simulink model "c00016M_harness"  (R2018a)
settings: Solver=FixedStepAuto  StartTime=0.0  StopTime=300  FixedStep=0.1  RelTol=1e-3
undefined symbols (not defined in the file): A1, hmax, PriorityTank, R1, R2, sigbuilder_block
(part 1 of 24)
settings Model: Creator=aarrieta  LastModifiedBy=umarkiegi

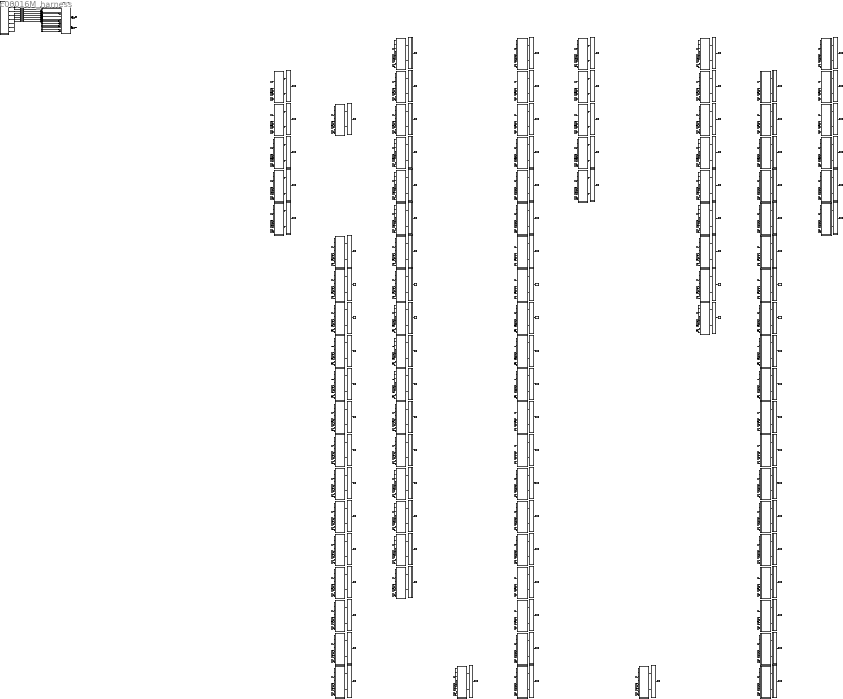
== system c00016M_harness ==
  CPSUT : Subsystem
  Eval100 : Subsystem
  Eval101 : Subsystem
  Eval102 : Subsystem
  Eval103 : Subsystem
  Eval104 : Subsystem
  Eval105 : Subsystem
  Eval106 : Subsystem
  Eval107 : Subsystem
  Eval108 : Subsystem
  Eval109 : Subsystem
  Eval110 : Subsystem
  Eval111 : Subsystem
  Eval112 : Subsystem
  Eval113 : Subsystem
  Eval114 : Subsystem
  Eval115 : Subsystem
  Eval116 : Subsystem
  Eval139 : Subsystem
  Eval140 : Subsystem
  Eval141 : Subsystem
  Eval142 : Subsystem
  Eval143 : Subsystem
  Eval144 : Subsystem
  Eval145 : Subsystem
  Eval146 : Subsystem
  Eval147 : Subsystem
  Eval148 : Subsystem
  Eval149 : Subsystem
  Eval150 : Subsystem
  Eval151 : Subsystem
  Eval152 : Subsystem
  Eval153 : Subsystem
  Eval154 : Subsystem
  Eval155 : Subsystem
  Eval156 : Subsystem
  Eval157 : Subsystem
  Eval158 : Subsystem
  Eval159 : Subsystem
  Eval160 : Subsystem
  Eval161 : Subsystem
  Eval162 : Subsystem
  Eval163 : Subsystem
  Eval164 : Subsystem
  Eval199 : Subsystem
  Eval200 : Subsystem
  Eval201 : Subsystem
  Eval202 : Subsystem
  Eval203 : Subsystem
  Eval204 : Subsystem
  Eval205 : Subsystem
  Eval206 : Subsystem
  Eval207 : Subsystem
  Eval208 : Subsystem
  Eval221 : Subsystem
  Eval222 : Subsystem
  Eval223 : Subsystem
  Eval224 : Subsystem
  Eval225 : Subsystem
  Eval226 : Subsystem
  Eval227 : Subsystem
  Eval228 : Subsystem
  Eval229 : Subsystem
  Eval230 : Subsystem
  Eval231 : Subsystem
  Eval232 : Subsystem
  Eval233 : Subsystem
  Eval234 : Subsystem
  Eval235 : Subsystem
  Eval236 : Subsystem
  Eval237 : Subsystem
  Eval238 : Subsystem
  Eval239 : Subsystem
  Eval240 : Subsystem
  Eval241 : Subsystem
  Eval242 : Subsystem
  Eval243 : Subsystem
  Eval244 : Subsystem
  Eval245 : Subsystem
  Eval61 : Subsystem
  Eval62 : Subsystem
  Eval63 : Subsystem
  Eval64 : Subsystem
  Eval65 : Subsystem
  Eval82 : Subsystem
  Eval86 : Subsystem
  Eval87 : Subsystem
  Eval88 : Subsystem
  Eval89 : Subsystem
  Eval90 : Subsystem
  Eval91 : Subsystem
  Eval92 : Subsystem
  Eval93 : Subsystem
  Eval94 : Subsystem
  Eval95 : Subsystem
  Eval96 : Subsystem
  Eval97 : Subsystem
  Eval98 : Subsystem
  Eval99 : Subsystem
  Inputs : Subsystem  Tag=STV Subsys  LoadFcn=sigbuilder_block('load');  StartFcn=sigbuilder_block('start');  StopFcn=sigbuilder_block('stop');  ClipboardFcn=sigbuilder_block('clipboard');  mask(Sigbuilder block){tuvar=[0:10]}
      mask init:
      | if ~strcmp(get_param(bdroot(gcb),'SimulationStatus'),'stopped'),tuvar = sigbuilder_block('maskInit'); end
      settings: CopyFcn=sigbuilder_block('copy');  DeleteFcn=sigbuilder_block('delete');  ModelCloseFcn=sigbuilder_block('modelClose');  PreSaveFcn=sigbuilder_block('preSave');  PauseFcn=sigbuilder_block('pause');  ContinueFcn=sigbuilder_block('continue');  NameChangeFcn=sigbuilder_block('namechange');  OpenFcn=sigbuilder_block('open',[276.75 163.5 675.75 486.75 ]);  CloseFcn=sigbuilder_block('close');
      mask Display: plot(0, 0, 100, 100,[2, 2, 32, 32, 2], [68, 8, 8, 68, 68],[32, 2], [38, 38], [32, 19, 2],[53, 60, 44], [32, 17, 17, 2],[16, 16, 31, 31]);txt = getActiveGroup(gcbh);text(2, 100, txt,'verticalAlignment', 'top');
  M062 : Subsystem
  M063 : Subsystem
  M064 : Subsystem
  M065 : Subsystem
  M066 : Subsystem
  M083 : Subsystem
  M087 : Subsystem
  M088 : Subsystem
  M089 : Subsystem
  M090 : Subsystem
  M091 : Subsystem
  M092 : Subsystem
  M093 : Subsystem
  M094 : Subsystem
  M095 : Subsystem
  M096 : Subsystem
  M097 : Subsystem
  M098 : Subsystem
  M099 : Subsystem
  M100 : Subsystem
  M101 : Subsystem
  M102 : Subsystem
  M103 : Subsystem
  M104 : Subsystem
  M105 : Subsystem
  M106 : Subsystem
  M107 : Subsystem
  M108 : Subsystem
  M109 : Subsystem
  M110 : Subsystem
  M111 : Subsystem
  M112 : Subsystem
  M113 : Subsystem
  M114 : Subsystem
  M115 : Subsystem
  M116 : Subsystem
  M117 : Subsystem
  M140 : Subsystem
  M141 : Subsystem
  M142 : Subsystem
  M143 : Subsystem
  M144 : Subsystem
  M145 : Subsystem
  M146 : Subsystem
  M147 : Subsystem
  M148 : Subsystem
  M149 : Subsystem
  M150 : Subsystem
  M151 : Subsystem
  M152 : Subsystem
  M153 : Subsystem
  M154 : Subsystem
  M155 : Subsystem
  M156 : Subsystem
  M157 : Subsystem
  M158 : Subsystem
  M159 : Subsystem
  M160 : Subsystem
  M161 : Subsystem
  M162 : Subsystem
  M163 : Subsystem
  M164 : Subsystem
  M165 : Subsystem
  M200 : Subsystem
  M201 : Subsystem
  M202 : Subsystem
  M203 : Subsystem
  M204 : Subsystem
  M205 : Subsystem
  M206 : Subsystem
  M207 : Subsystem
  M208 : Subsystem
  M209 : Subsystem
  M222 : Subsystem
  M223 : Subsystem
  M224 : Subsystem
  M225 : Subsystem
  M226 : Subsystem
  M227 : Subsystem
  M228 : Subsystem
  M229 : Subsystem
  M230 : Subsystem
  M231 : Subsystem
  M232 : Subsystem
  M233 : Subsystem
  M234 : Subsystem
  M235 : Subsystem
  M236 : Subsystem
  M237 : Subsystem
  M238 : Subsystem
  M239 : Subsystem
  M240 : Subsystem
  M241 : Subsystem
  M242 : Subsystem
  M243 : Subsystem
  M244 : Subsystem
  M245 : Subsystem
  M246 : Subsystem
  To Workspace100 : ToWorkspace  VariableName=mutant101  SampleTime=-1
  To Workspace101 : ToWorkspace  VariableName=mutant102  SampleTime=-1
  To Workspace102 : ToWorkspace  VariableName=mutant103  SampleTime=-1
  To Workspace103 : ToWorkspace  VariableName=mutant104  SampleTime=-1
  To Workspace104 : ToWorkspace  VariableName=mutant105  SampleTime=-1
  To Workspace105 : ToWorkspace  VariableName=mutant106  SampleTime=-1
  To Workspace106 : ToWorkspace  VariableName=mutant107  SampleTime=-1
  To Workspace107 : ToWorkspace  VariableName=mutant108  SampleTime=-1
  To Workspace108 : ToWorkspace  VariableName=mutant109  SampleTime=-1
  To Workspace109 : ToWorkspace  VariableName=mutant110  SampleTime=-1
  To Workspace110 : ToWorkspace  VariableName=mutant111  SampleTime=-1
  To Workspace111 : ToWorkspace  VariableName=mutant112  SampleTime=-1
  To Workspace112 : ToWorkspace  VariableName=mutant113  SampleTime=-1
  To Workspace113 : ToWorkspace  VariableName=mutant114  SampleTime=-1
  To Workspace114 : ToWorkspace  VariableName=mutant115  SampleTime=-1
  To Workspace115 : ToWorkspace  VariableName=mutant116  SampleTime=-1
  To Workspace116 : ToWorkspace  VariableName=mutant117  SampleTime=-1
  To Workspace139 : ToWorkspace  VariableName=mutant140  SampleTime=-1
  To Workspace140 : ToWorkspace  VariableName=mutant141  SampleTime=-1
  To Workspace141 : ToWorkspace  VariableName=mutant142  SampleTime=-1
  To Workspace142 : ToWorkspace  VariableName=mutant143  SampleTime=-1
  To Workspace143 : ToWorkspace  VariableName=mutant144  SampleTime=-1
  To Workspace144 : ToWorkspace  VariableName=mutant145  SampleTime=-1
  To Workspace145 : ToWorkspace  VariableName=mutant146  SampleTime=-1
  To Workspace146 : ToWorkspace  VariableName=mutant147  SampleTime=-1
  To Workspace147 : ToWorkspace  VariableName=mutant148  SampleTime=-1
  To Workspace148 : ToWorkspace  VariableName=mutant149  SampleTime=-1
  To Workspace149 : ToWorkspace  VariableName=mutant150  SampleTime=-1
  To Workspace150 : ToWorkspace  VariableName=mutant151  SampleTime=-1
  To Workspace151 : ToWorkspace  VariableName=mutant152  SampleTime=-1
  To Workspace152 : ToWorkspace  VariableName=mutant153  SampleTime=-1
  To Workspace153 : ToWorkspace  VariableName=mutant154  SampleTime=-1
  To Workspace154 : ToWorkspace  VariableName=mutant155  SampleTime=-1
  To Workspace155 : ToWorkspace  VariableName=mutant156  SampleTime=-1
  To Workspace156 : ToWorkspace  VariableName=mutant157  SampleTime=-1
  To Workspace157 : ToWorkspace  VariableName=mutant158  SampleTime=-1
  To Workspace158 : ToWorkspace  VariableName=mutant159  SampleTime=-1
  To Workspace159 : ToWorkspace  VariableName=mutant160  SampleTime=-1
  To Workspace160 : ToWorkspace  VariableName=mutant161  SampleTime=-1
  To Workspace161 : ToWorkspace  VariableName=mutant162  SampleTime=-1
  To Workspace162 : ToWorkspace  VariableName=mutant163  SampleTime=-1
  To Workspace163 : ToWorkspace  VariableName=mutant164  SampleTime=-1
  To Workspace164 : ToWorkspace  VariableName=mutant165  SampleTime=-1
  To Workspace199 : ToWorkspace  VariableName=mutant200  SampleTime=-1
  To Workspace200 : ToWorkspace  VariableName=mutant201  SampleTime=-1
  To Workspace201 : ToWorkspace  VariableName=mutant202  SampleTime=-1
  To Workspace202 : ToWorkspace  VariableName=mutant203  SampleTime=-1
  To Workspace203 : ToWorkspace  VariableName=mutant204  SampleTime=-1
  To Workspace204 : ToWorkspace  VariableName=mutant205  SampleTime=-1
  To Workspace205 : ToWorkspace  VariableName=mutant206  SampleTime=-1
  To Workspace206 : ToWorkspace  VariableName=mutant207  SampleTime=-1
  To Workspace207 : ToWorkspace  VariableName=mutant208  SampleTime=-1
  To Workspace208 : ToWorkspace  VariableName=mutant209  SampleTime=-1
  To Workspace221 : ToWorkspace  VariableName=mutant222  SampleTime=-1
  To Workspace222 : ToWorkspace  VariableName=mutant223  SampleTime=-1
  To Workspace223 : ToWorkspace  VariableName=mutant224  SampleTime=-1
  To Workspace224 : ToWorkspace  VariableName=mutant225  SampleTime=-1
  To Workspace225 : ToWorkspace  VariableName=mutant226  SampleTime=-1
  To Workspace226 : ToWorkspace  VariableName=mutant227  SampleTime=-1
  To Workspace227 : ToWorkspace  VariableName=mutant228  SampleTime=-1
  To Workspace228 : ToWorkspace  VariableName=mutant229  SampleTime=-1
  To Workspace229 : ToWorkspace  VariableName=mutant230  SampleTime=-1
  To Workspace230 : ToWorkspace  VariableName=mutant231  SampleTime=-1
  To Workspace231 : ToWorkspace  VariableName=mutant232  SampleTime=-1
  To Workspace232 : ToWorkspace  VariableName=mutant233  SampleTime=-1
  To Workspace233 : ToWorkspace  VariableName=mutant234  SampleTime=-1
  To Workspace234 : ToWorkspace  VariableName=mutant235  SampleTime=-1
  To Workspace235 : ToWorkspace  VariableName=mutant236  SampleTime=-1
  To Workspace236 : ToWorkspace  VariableName=mutant237  SampleTime=-1
  To Workspace237 : ToWorkspace  VariableName=mutant238  SampleTime=-1
  To Workspace238 : ToWorkspace  VariableName=mutant239  SampleTime=-1
  To Workspace239 : ToWorkspace  VariableName=mutant240  SampleTime=-1
  To Workspace240 : ToWorkspace  VariableName=mutant241  SampleTime=-1
  To Workspace241 : ToWorkspace  VariableName=mutant242  SampleTime=-1
  To Workspace242 : ToWorkspace  VariableName=mutant243  SampleTime=-1
  To Workspace243 : ToWorkspace  VariableName=mutant244  SampleTime=-1
  To Workspace244 : ToWorkspace  VariableName=mutant245  SampleTime=-1
  To Workspace245 : ToWorkspace  VariableName=mutant246  SampleTime=-1
  To Workspace61 : ToWorkspace  VariableName=mutant062  SampleTime=-1
  To Workspace62 : ToWorkspace  VariableName=mutant063  SampleTime=-1
  To Workspace63 : ToWorkspace  VariableName=mutant064  SampleTime=-1
  To Workspace64 : ToWorkspace  VariableName=mutant065  SampleTime=-1
  To Workspace65 : ToWorkspace  VariableName=mutant066  SampleTime=-1
  To Workspace82 : ToWorkspace  VariableName=mutant083  SampleTime=-1
  To Workspace86 : ToWorkspace  VariableName=mutant087  SampleTime=-1
  To Workspace87 : ToWorkspace  VariableName=mutant088  SampleTime=-1
  To Workspace88 : ToWorkspace  VariableName=mutant089  SampleTime=-1
  To Workspace89 : ToWorkspace  VariableName=mutant090  SampleTime=-1
  To Workspace90 : ToWorkspace  VariableName=mutant091  SampleTime=-1
  To Workspace91 : ToWorkspace  VariableName=mutant092  SampleTime=-1
  To Workspace92 : ToWorkspace  VariableName=mutant093  SampleTime=-1
  To Workspace93 : ToWorkspace  VariableName=mutant094  SampleTime=-1
  To Workspace94 : ToWorkspace  VariableName=mutant095  SampleTime=-1
  To Workspace95 : ToWorkspace  VariableName=mutant096  SampleTime=-1
  To Workspace96 : ToWorkspace  VariableName=mutant097  SampleTime=-1
  To Workspace97 : ToWorkspace  VariableName=mutant098  SampleTime=-1
  To Workspace98 : ToWorkspace  VariableName=mutant099  SampleTime=-1
  To Workspace99 : ToWorkspace  VariableName=mutant100  SampleTime=-1
  dtc_CT2 : DataTypeConversion
  dtc_CT3 : DataTypeConversion
  dtc_E3 : DataTypeConversion
  dtc_EB2 : DataTypeConversion
  dtc_EB3 : DataTypeConversion
  dtc_F3 : DataTypeConversion
  dtc_T2 : DataTypeConversion
  dtc_T3 : DataTypeConversion
  LL2 : Outport
  LL3 : Outport  Port=2
  tag scope: out2=global, out3=global
  wires:
  CPSUT/1(LL2) -> [out2], LL2/1
  CPSUT/2(LL3) -> [out3], LL3/1
  [in7] -> M062/1(CT2)
  [in11] -> M062/2(T2)
  [in12] -> M062/3(EB2)
  [in13] -> M062/4(CT3)
  [in14] -> M062/5(F3)
  [in15] -> M062/6(E3)
  [in17] -> M062/7(T3)
  [in18] -> M062/8(EB3)
  M062/1(LL2) -> Eval61/1(In2)
  M062/2(LL3) -> Eval61/2(In3)
  Eval61/1(Out1) -> To Workspace61/1
  [in7] -> M063/1(CT2)
  [in11] -> M063/2(T2)
  [in12] -> M063/3(EB2)
  [in13] -> M063/4(CT3)
  [in14] -> M063/5(F3)
  [in15] -> M063/6(E3)
  [in17] -> M063/7(T3)
  [in18] -> M063/8(EB3)
  M063/1(LL2) -> Eval62/1(In2)
  M063/2(LL3) -> Eval62/2(In3)
  Eval62/1(Out1) -> To Workspace62/1
  [in7] -> M064/1(CT2)
  [in11] -> M064/2(T2)
  [in12] -> M064/3(EB2)
  [in13] -> M064/4(CT3)
  [in14] -> M064/5(F3)
  [in15] -> M064/6(E3)
  [in17] -> M064/7(T3)
  [in18] -> M064/8(EB3)
  M064/1(LL2) -> Eval63/1(In2)
  M064/2(LL3) -> Eval63/2(In3)
  Eval63/1(Out1) -> To Workspace63/1
  [in7] -> M065/1(CT2)
  [in11] -> M065/2(T2)
  [in12] -> M065/3(EB2)
  [in13] -> M065/4(CT3)
  [in14] -> M065/5(F3)
  [in15] -> M065/6(E3)
  [in17] -> M065/7(T3)
  [in18] -> M065/8(EB3)
  M065/1(LL2) -> Eval64/1(In2)
  M065/2(LL3) -> Eval64/2(In3)
  Eval64/1(Out1) -> To Workspace64/1
  [in7] -> M066/1(CT2)
  [in11] -> M066/2(T2)
  [in12] -> M066/3(EB2)
  [in13] -> M066/4(CT3)
  [in14] -> M066/5(F3)
  [in15] -> M066/6(E3)
  [in17] -> M066/7(T3)
  [in18] -> M066/8(EB3)
  M066/1(LL2) -> Eval65/1(In2)
  M066/2(LL3) -> Eval65/2(In3)
  Eval65/1(Out1) -> To Workspace65/1
  [in7] -> M083/1(CT2)
  [in11] -> M083/2(T2)
  [in12] -> M083/3(EB2)
  [in13] -> M083/4(CT3)
  [in14] -> M083/5(F3)
  [in15] -> M083/6(E3)
  [in17] -> M083/7(T3)
  [in18] -> M083/8(EB3)
  M083/1(LL2) -> Eval82/1(In2)
  M083/2(LL3) -> Eval82/2(In3)
  Eval82/1(Out1) -> To Workspace82/1
  [in7] -> M087/1(CT2)
  [in11] -> M087/2(T2)
  [in12] -> M087/3(EB2)
  [in13] -> M087/4(CT3)
  [in14] -> M087/5(F3)
  [in15] -> M087/6(E3)
  [in17] -> M087/7(T3)
  [in18] -> M087/8(EB3)
  M087/1(LL2) -> Eval86/1(In2)
  M087/2(LL3) -> Eval86/2(In3)
  Eval86/1(Out1) -> To Workspace86/1
  [in7] -> M088/1(CT2)
  [in11] -> M088/2(T2)
  [in12] -> M088/3(EB2)
  [in13] -> M088/4(CT3)
  [in14] -> M088/5(F3)
  [in15] -> M088/6(E3)
  [in17] -> M088/7(T3)
  [in18] -> M088/8(EB3)
  M088/1(LL2) -> Eval87/1(In2)
  M088/2(LL3) -> Eval87/2(In3)
  Eval87/1(Out1) -> To Workspace87/1
  [in7] -> M089/1(CT2)
  [in11] -> M089/2(T2)
  [in12] -> M089/3(EB2)
  [in13] -> M089/4(CT3)
  [in14] -> M089/5(F3)
  [in15] -> M089/6(E3)
  [in17] -> M089/7(T3)
  [in18] -> M089/8(EB3)
  M089/1(LL2) -> Eval88/1(In2)
  M089/2(LL3) -> Eval88/2(In3)
  Eval88/1(Out1) -> To Workspace88/1
  [in7] -> M090/1(CT2)
  [in11] -> M090/2(T2)
  [in12] -> M090/3(EB2)
  [in13] -> M090/4(CT3)
  [in14] -> M090/5(F3)
  [in15] -> M090/6(E3)
  [in17] -> M090/7(T3)
  [in18] -> M090/8(EB3)
  M090/1(LL2) -> Eval89/1(In2)
  M090/2(LL3) -> Eval89/2(In3)
  Eval89/1(Out1) -> To Workspace89/1
  [in7] -> M091/1(CT2)
  [in11] -> M091/2(T2)
  [in12] -> M091/3(EB2)
  [in13] -> M091/4(CT3)
  [in14] -> M091/5(F3)
  [in15] -> M091/6(E3)
  [in17] -> M091/7(T3)
  [in18] -> M091/8(EB3)
  M091/1(LL2) -> Eval90/1(In2)
  M091/2(LL3) -> Eval90/2(In3)
  Eval90/1(Out1) -> To Workspace90/1
  [in7] -> M092/1(CT2)
  [in11] -> M092/2(T2)
  [in12] -> M092/3(EB2)
  [in13] -> M092/4(CT3)
  [in14] -> M092/5(F3)
  [in15] -> M092/6(E3)
  [in17] -> M092/7(T3)
  [in18] -> M092/8(EB3)
  M092/1(LL2) -> Eval91/1(In2)
  M092/2(LL3) -> Eval91/2(In3)
  Eval91/1(Out1) -> To Workspace91/1
  [in7] -> M093/1(CT2)
  [in11] -> M093/2(T2)
  [in12] -> M093/3(EB2)
  [in13] -> M093/4(CT3)
  [in14] -> M093/5(F3)
  [in15] -> M093/6(E3)
  [in17] -> M093/7(T3)
  [in18] -> M093/8(EB3)
  M093/1(LL2) -> Eval92/1(In2)
  M093/2(LL3) -> Eval92/2(In3)
  Eval92/1(Out1) -> To Workspace92/1
  [in7] -> M094/1(CT2)
  [in11] -> M094/2(T2)
  [in12] -> M094/3(EB2)
  [in13] -> M094/4(CT3)
  [in14] -> M094/5(F3)
  [in15] -> M094/6(E3)
  [in17] -> M094/7(T3)
  [in18] -> M094/8(EB3)
  M094/1(LL2) -> Eval93/1(In2)
  M094/2(LL3) -> Eval93/2(In3)
  Eval93/1(Out1) -> To Workspace93/1
  [in7] -> M095/1(CT2)
  [in11] -> M095/2(T2)
  [in12] -> M095/3(EB2)
  [in13] -> M095/4(CT3)
  [in14] -> M095/5(F3)
  [in15] -> M095/6(E3)
  [in17] -> M095/7(T3)
  [in18] -> M095/8(EB3)
  M095/1(LL2) -> Eval94/1(In2)
  M095/2(LL3) -> Eval94/2(In3)
  Eval94/1(Out1) -> To Workspace94/1
  [in7] -> M096/1(CT2)
  [in11] -> M096/2(T2)
  [in12] -> M096/3(EB2)
  [in13] -> M096/4(CT3)
  [in14] -> M096/5(F3)
  [in15] -> M096/6(E3)
  [in17] -> M096/7(T3)
  [in18] -> M096/8(EB3)
  M096/1(LL2) -> Eval95/1(In2)
  M096/2(LL3) -> Eval95/2(In3)
  Eval95/1(Out1) -> To Workspace95/1
  [in7] -> M097/1(CT2)
  [in11] -> M097/2(T2)
  [in12] -> M097/3(EB2)
  [in13] -> M097/4(CT3)
  [in14] -> M097/5(F3)
  [in15] -> M097/6(E3)
  [in17] -> M097/7(T3)
  [in18] -> M097/8(EB3)
  M097/1(LL2) -> Eval96/1(In2)
  M097/2(LL3) -> Eval96/2(In3)
  Eval96/1(Out1) -> To Workspace96/1
  [in7] -> M098/1(CT2)
  [in11] -> M098/2(T2)
  [in12] -> M098/3(EB2)
  [in13] -> M098/4(CT3)
  [in14] -> M098/5(F3)
  [in15] -> M098/6(E3)
  [in17] -> M098/7(T3)
  [in18] -> M098/8(EB3)
  M098/1(LL2) -> Eval97/1(In2)
  M098/2(LL3) -> Eval97/2(In3)
  Eval97/1(Out1) -> To Workspace97/1
  [in7] -> M099/1(CT2)
  [in11] -> M099/2(T2)
  [in12] -> M099/3(EB2)
  [in13] -> M099/4(CT3)
  [in14] -> M099/5(F3)
  [in15] -> M099/6(E3)
  [in17] -> M099/7(T3)
  [in18] -> M099/8(EB3)
  M099/1(LL2) -> Eval98/1(In2)
  M099/2(LL3) -> Eval98/2(In3)
  Eval98/1(Out1) -> To Workspace98/1
  [in7] -> M100/1(CT2)
  [in11] -> M100/2(T2)
  [in12] -> M100/3(EB2)
  [in13] -> M100/4(CT3)
  [in14] -> M100/5(F3)
  [in15] -> M100/6(E3)
  [in17] -> M100/7(T3)
  [in18] -> M100/8(EB3)
  M100/1(LL2) -> Eval99/1(In2)
  M100/2(LL3) -> Eval99/2(In3)
  Eval99/1(Out1) -> To Workspace99/1
  [in7] -> M101/1(CT2)
  [in11] -> M101/2(T2)
  [in12] -> M101/3(EB2)
  [in13] -> M101/4(CT3)
  [in14] -> M101/5(F3)
  [in15] -> M101/6(E3)
  [in17] -> M101/7(T3)
  [in18] -> M101/8(EB3)
  M101/1(LL2) -> Eval100/1(In2)
  M101/2(LL3) -> Eval100/2(In3)
  Eval100/1(Out1) -> To Workspace100/1
  [in7] -> M102/1(CT2)
  [in11] -> M102/2(T2)
  [in12] -> M102/3(EB2)
  [in13] -> M102/4(CT3)
  [in14] -> M102/5(F3)
  [in15] -> M102/6(E3)
  [in17] -> M102/7(T3)
  [in18] -> M102/8(EB3)
  M102/1(LL2) -> Eval101/1(In2)
  M102/2(LL3) -> Eval101/2(In3)
  Eval101/1(Out1) -> To Workspace101/1
  [in7] -> M103/1(CT2)
  [in11] -> M103/2(T2)
  [in12] -> M103/3(EB2)
  [in13] -> M103/4(CT3)
  [in14] -> M103/5(F3)
  [in15] -> M103/6(E3)
  [in17] -> M103/7(T3)
  [in18] -> M103/8(EB3)
  M103/1(LL2) -> Eval102/1(In2)
  M103/2(LL3) -> Eval102/2(In3)
  Eval102/1(Out1) -> To Workspace102/1
  [in7] -> M104/1(CT2)
  [in11] -> M104/2(T2)
  [in12] -> M104/3(EB2)
  [in13] -> M104/4(CT3)
  [in14] -> M104/5(F3)
  [in15] -> M104/6(E3)
  [in17] -> M104/7(T3)
  [in18] -> M104/8(EB3)
  M104/1(LL2) -> Eval103/1(In2)
  M104/2(LL3) -> Eval103/2(In3)
  Eval103/1(Out1) -> To Workspace103/1
  [in7] -> M105/1(CT2)
  [in11] -> M105/2(T2)
  [in12] -> M105/3(EB2)
  [in13] -> M105/4(CT3)
  [in14] -> M105/5(F3)
  [in15] -> M105/6(E3)
  [in17] -> M105/7(T3)
  [in18] -> M105/8(EB3)
  M105/1(LL2) -> Eval104/1(In2)
  M105/2(LL3) -> Eval104/2(In3)
  Eval104/1(Out1) -> To Workspace104/1
  [in7] -> M106/1(CT2)
  [in11] -> M106/2(T2)
  [in12] -> M106/3(EB2)
  [in13] -> M106/4(CT3)
  [in14] -> M106/5(F3)
  [in15] -> M106/6(E3)
  [in17] -> M106/7(T3)
  [in18] -> M106/8(EB3)
  M106/1(LL2) -> Eval105/1(In2)
  M106/2(LL3) -> Eval105/2(In3)
  Eval105/1(Out1) -> To Workspace105/1
  [in7] -> M107/1(CT2)
  [in11] -> M107/2(T2)
  [in12] -> M107/3(EB2)
  [in13] -> M107/4(CT3)
  [in14] -> M107/5(F3)
  [in15] -> M107/6(E3)
  [in17] -> M107/7(T3)
  [in18] -> M107/8(EB3)
  M107/1(LL2) -> Eval106/1(In2)
  M107/2(LL3) -> Eval106/2(In3)
  Eval106/1(Out1) -> To Workspace106/1
  [in7] -> M108/1(CT2)
  [in11] -> M108/2(T2)
  [in12] -> M108/3(EB2)
  [in13] -> M108/4(CT3)
  [in14] -> M108/5(F3)
  [in15] -> M108/6(E3)
  [in17] -> M108/7(T3)
  [in18] -> M108/8(EB3)
  M108/1(LL2) -> Eval107/1(In2)
  M108/2(LL3) -> Eval107/2(In3)
  Eval107/1(Out1) -> To Workspace107/1
  [in7] -> M109/1(CT2)
  [in11] -> M109/2(T2)
  [in12] -> M109/3(EB2)
  [in13] -> M109/4(CT3)
  [in14] -> M109/5(F3)
  [in15] -> M109/6(E3)
  [in17] -> M109/7(T3)
  [in18] -> M109/8(EB3)
  M109/1(LL2) -> Eval108/1(In2)
  M109/2(LL3) -> Eval108/2(In3)
  Eval108/1(Out1) -> To Workspace108/1
  [in7] -> M110/1(CT2)
  [in11] -> M110/2(T2)
  [in12] -> M110/3(EB2)
  [in13] -> M110/4(CT3)
  [in14] -> M110/5(F3)
  [in15] -> M110/6(E3)
  [in17] -> M110/7(T3)
  [in18] -> M110/8(EB3)
  M110/1(LL2) -> Eval109/1(In2)
  M110/2(LL3) -> Eval109/2(In3)
  Eval109/1(Out1) -> To Workspace109/1
  [in7] -> M111/1(CT2)
  [in11] -> M111/2(T2)
  [in12] -> M111/3(EB2)
  [in13] -> M111/4(CT3)
  [in14] -> M111/5(F3)
  [in15] -> M111/6(E3)
  [in17] -> M111/7(T3)
  [in18] -> M111/8(EB3)
  M111/1(LL2) -> Eval110/1(In2)
  M111/2(LL3) -> Eval110/2(In3)
  Eval110/1(Out1) -> To Workspace110/1
  [in7] -> M112/1(CT2)
  [in11] -> M112/2(T2)
  [in12] -> M112/3(EB2)
  [in13] -> M112/4(CT3)
  [in14] -> M112/5(F3)
  [in15] -> M112/6(E3)
  [in17] -> M112/7(T3)
  [in18] -> M112/8(EB3)
  M112/1(LL2) -> Eval111/1(In2)
  M112/2(LL3) -> Eval111/2(In3)
  Eval111/1(Out1) -> To Workspace111/1
  [in7] -> M113/1(CT2)
  [in11] -> M113/2(T2)
  [in12] -> M113/3(EB2)
  [in13] -> M113/4(CT3)
  [in14] -> M113/5(F3)
  [in15] -> M113/6(E3)
  [in17] -> M113/7(T3)
  [in18] -> M113/8(EB3)
  M113/1(LL2) -> Eval112/1(In2)
  M113/2(LL3) -> Eval112/2(In3)
  Eval112/1(Out1) -> To Workspace112/1
  [in7] -> M114/1(CT2)
  [in11] -> M114/2(T2)
  [in12] -> M114/3(EB2)
  [in13] -> M114/4(CT3)
  [in14] -> M114/5(F3)
  [in15] -> M114/6(E3)
  [in17] -> M114/7(T3)
  [in18] -> M114/8(EB3)
  M114/1(LL2) -> Eval113/1(In2)
  M114/2(LL3) -> Eval113/2(In3)
  Eval113/1(Out1) -> To Workspace113/1
  [in7] -> M115/1(CT2)
  [in11] -> M115/2(T2)
  [in12] -> M115/3(EB2)
  [in13] -> M115/4(CT3)
  [in14] -> M115/5(F3)
  [in15] -> M115/6(E3)
  [in17] -> M115/7(T3)
  [in18] -> M115/8(EB3)
  M115/1(LL2) -> Eval114/1(In2)
  M115/2(LL3) -> Eval114/2(In3)
  Eval114/1(Out1) -> To Workspace114/1
  [in7] -> M116/1(CT2)
  [in11] -> M116/2(T2)
  [in12] -> M116/3(EB2)
  [in13] -> M116/4(CT3)
  [in14] -> M116/5(F3)
  [in15] -> M116/6(E3)
  [in17] -> M116/7(T3)
  [in18] -> M116/8(EB3)
  M116/1(LL2) -> Eval115/1(In2)
  M116/2(LL3) -> Eval115/2(In3)
  Eval115/1(Out1) -> To Workspace115/1
  [in7] -> M117/1(CT2)
  [in11] -> M117/2(T2)
  [in12] -> M117/3(EB2)
  [in13] -> M117/4(CT3)
  [in14] -> M117/5(F3)
  [in15] -> M117/6(E3)
  [in17] -> M117/7(T3)
  [in18] -> M117/8(EB3)
  M117/1(LL2) -> Eval116/1(In2)
  M117/2(LL3) -> Eval116/2(In3)
  Eval116/1(Out1) -> To Workspace116/1
  [in7] -> M140/1(CT2)
  [in11] -> M140/2(T2)
  [in12] -> M140/3(EB2)
  [in13] -> M140/4(CT3)
  [in14] -> M140/5(F3)
  [in15] -> M140/6(E3)
  [in17] -> M140/7(T3)
  [in18] -> M140/8(EB3)
  M140/1(LL2) -> Eval139/1(In2)
  M140/2(LL3) -> Eval139/2(In3)
  Eval139/1(Out1) -> To Workspace139/1
  [in7] -> M141/1(CT2)
  [in11] -> M141/2(T2)
  [in12] -> M141/3(EB2)
  [in13] -> M141/4(CT3)
  [in14] -> M141/5(F3)
  [in15] -> M141/6(E3)
  [in17] -> M141/7(T3)
  [in18] -> M141/8(EB3)
  M141/1(LL2) -> Eval140/1(In2)
  M141/2(LL3) -> Eval140/2(In3)
  Eval140/1(Out1) -> To Workspace140/1
  [in7] -> M142/1(CT2)
  [in11] -> M142/2(T2)
  [in12] -> M142/3(EB2)
  [in13] -> M142/4(CT3)
  [in14] -> M142/5(F3)
  [in15] -> M142/6(E3)
  [in17] -> M142/7(T3)
  [in18] -> M142/8(EB3)
  M142/1(LL2) -> Eval141/1(In2)
  M142/2(LL3) -> Eval141/2(In3)
  Eval141/1(Out1) -> To Workspace141/1
  [in7] -> M143/1(CT2)
  [in11] -> M143/2(T2)
  [in12] -> M143/3(EB2)
  [in13] -> M143/4(CT3)
  [in14] -> M143/5(F3)
  [in15] -> M143/6(E3)
  [in17] -> M143/7(T3)
  [in18] -> M143/8(EB3)
  M143/1(LL2) -> Eval142/1(In2)
  M143/2(LL3) -> Eval142/2(In3)
  Eval142/1(Out1) -> To Workspace142/1
  [in7] -> M144/1(CT2)
  [in11] -> M144/2(T2)
  [in12] -> M144/3(EB2)
  [in13] -> M144/4(CT3)
  [in14] -> M144/5(F3)
  [in15] -> M144/6(E3)
  [in17] -> M144/7(T3)
  [in18] -> M144/8(EB3)
  M144/1(LL2) -> Eval143/1(In2)
  M144/2(LL3) -> Eval143/2(In3)
  Eval143/1(Out1) -> To Workspace143/1
  [in7] -> M145/1(CT2)
  [in11] -> M145/2(T2)
  [in12] -> M145/3(EB2)
  [in13] -> M145/4(CT3)
  [in14] -> M145/5(F3)
  [in15] -> M145/6(E3)
  [in17] -> M145/7(T3)
  [in18] -> M145/8(EB3)
  M145/1(LL2) -> Eval144/1(In2)
  M145/2(LL3) -> Eval144/2(In3)
  Eval144/1(Out1) -> To Workspace144/1
  [in7] -> M146/1(CT2)
  [in11] -> M146/2(T2)
  [in12] -> M146/3(EB2)
  [in13] -> M146/4(CT3)
  [in14] -> M146/5(F3)
  [in15] -> M146/6(E3)
  [in17] -> M146/7(T3)
  [in18] -> M146/8(EB3)
  M146/1(LL2) -> Eval145/1(In2)
  M146/2(LL3) -> Eval145/2(In3)
  Eval145/1(Out1) -> To Workspace145/1
  [in7] -> M147/1(CT2)
  [in11] -> M147/2(T2)
  [in12] -> M147/3(EB2)
  [in13] -> M147/4(CT3)
  [in14] -> M147/5(F3)
  [in15] -> M147/6(E3)
  [in17] -> M147/7(T3)
  [in18] -> M147/8(EB3)
  M147/1(LL2) -> Eval146/1(In2)
  M147/2(LL3) -> Eval146/2(In3)
  Eval146/1(Out1) -> To Workspace146/1
  [in7] -> M148/1(CT2)
  [in11] -> M148/2(T2)
  [in12] -> M148/3(EB2)
  [in13] -> M148/4(CT3)
  [in14] -> M148/5(F3)
  [in15] -> M148/6(E3)
  [in17] -> M148/7(T3)
  [in18] -> M148/8(EB3)
  M148/1(LL2) -> Eval147/1(In2)
  M148/2(LL3) -> Eval147/2(In3)
  Eval147/1(Out1) -> To Workspace147/1
  [in7] -> M149/1(CT2)
  [in11] -> M149/2(T2)
  [in12] -> M149/3(EB2)
  [in13] -> M149/4(CT3)
  [in14] -> M149/5(F3)
  [in15] -> M149/6(E3)
  [in17] -> M149/7(T3)
  [in18] -> M149/8(EB3)
  M149/1(LL2) -> Eval148/1(In2)
  M149/2(LL3) -> Eval148/2(In3)
  Eval148/1(Out1) -> To Workspace148/1
  [in7] -> M150/1(CT2)
  [in11] -> M150/2(T2)
  [in12] -> M150/3(EB2)
  [in13] -> M150/4(CT3)
  [in14] -> M150/5(F3)
  [in15] -> M150/6(E3)
  [in17] -> M150/7(T3)
  [in18] -> M150/8(EB3)
  M150/1(LL2) -> Eval149/1(In2)
  M150/2(LL3) -> Eval149/2(In3)
  Eval149/1(Out1) -> To Workspace149/1
  [in7] -> M151/1(CT2)
  [in11] -> M151/2(T2)
  [in12] -> M151/3(EB2)
  [in13] -> M151/4(CT3)
  [in14] -> M151/5(F3)
  [in15] -> M151/6(E3)
  [in17] -> M151/7(T3)
  [in18] -> M151/8(EB3)
  M151/1(LL2) -> Eval150/1(In2)
  M151/2(LL3) -> Eval150/2(In3)
  Eval150/1(Out1) -> To Workspace150/1
  [in7] -> M152/1(CT2)
  [in11] -> M152/2(T2)
  [in12] -> M152/3(EB2)
  [in13] -> M152/4(CT3)
  [in14] -> M152/5(F3)
  [in15] -> M152/6(E3)
  [in17] -> M152/7(T3)
  [in18] -> M152/8(EB3)
  M152/1(LL2) -> Eval151/1(In2)
  M152/2(LL3) -> Eval151/2(In3)
  Eval151/1(Out1) -> To Workspace151/1
  [in7] -> M153/1(CT2)
  [in11] -> M153/2(T2)
  [in12] -> M153/3(EB2)
  [in13] -> M153/4(CT3)
  [in14] -> M153/5(F3)
  [in15] -> M153/6(E3)
  [in17] -> M153/7(T3)
  [in18] -> M153/8(EB3)
  M153/1(LL2) -> Eval152/1(In2)
  M153/2(LL3) -> Eval152/2(In3)
  Eval152/1(Out1) -> To Workspace152/1
  [in7] -> M154/1(CT2)
  [in11] -> M154/2(T2)
  [in12] -> M154/3(EB2)
  [in13] -> M154/4(CT3)
  [in14] -> M154/5(F3)
  [in15] -> M154/6(E3)
  [in17] -> M154/7(T3)
  [in18] -> M154/8(EB3)
  M154/1(LL2) -> Eval153/1(In2)
  M154/2(LL3) -> Eval153/2(In3)
  Eval153/1(Out1) -> To Workspace153/1
  [in7] -> M155/1(CT2)
  [in11] -> M155/2(T2)
  [in12] -> M155/3(EB2)
  [in13] -> M155/4(CT3)
  [in14] -> M155/5(F3)
  [in15] -> M155/6(E3)
  [in17] -> M155/7(T3)
  [in18] -> M155/8(EB3)
  M155/1(LL2) -> Eval154/1(In2)
  M155/2(LL3) -> Eval154/2(In3)
  Eval154/1(Out1) -> To Workspace154/1
  [in7] -> M156/1(CT2)
  [in11] -> M156/2(T2)
  [in12] -> M156/3(EB2)
  [in13] -> M156/4(CT3)
  [in14] -> M156/5(F3)
  [in15] -> M156/6(E3)
  [in17] -> M156/7(T3)
  [in18] -> M156/8(EB3)
  M156/1(LL2) -> Eval155/1(In2)
  M156/2(LL3) -> Eval155/2(In3)
  Eval155/1(Out1) -> To Workspace155/1
  [in7] -> M157/1(CT2)
  [in11] -> M157/2(T2)
  [in12] -> M157/3(EB2)
  [in13] -> M157/4(CT3)
  [in14] -> M157/5(F3)
  [in15] -> M157/6(E3)
  [in17] -> M157/7(T3)
  [in18] -> M157/8(EB3)
  M157/1(LL2) -> Eval156/1(In2)
  M157/2(LL3) -> Eval156/2(In3)
  Eval156/1(Out1) -> To Workspace156/1
  [in7] -> M158/1(CT2)
  [in11] -> M158/2(T2)
  [in12] -> M158/3(EB2)
  [in13] -> M158/4(CT3)
  [in14] -> M158/5(F3)
  [in15] -> M158/6(E3)
  [in17] -> M158/7(T3)
  [in18] -> M158/8(EB3)
  M158/1(LL2) -> Eval157/1(In2)
  M158/2(LL3) -> Eval157/2(In3)
  Eval157/1(Out1) -> To Workspace157/1
  [in7] -> M159/1(CT2)
  [in11] -> M159/2(T2)
  [in12] -> M159/3(EB2)
  [in13] -> M159/4(CT3)
  [in14] -> M159/5(F3)
  [in15] -> M159/6(E3)
  [in17] -> M159/7(T3)
  [in18] -> M159/8(EB3)
  M159/1(LL2) -> Eval158/1(In2)
  M159/2(LL3) -> Eval158/2(In3)
  Eval158/1(Out1) -> To Workspace158/1
  [in7] -> M160/1(CT2)
  [in11] -> M160/2(T2)
  [in12] -> M160/3(EB2)
  [in13] -> M160/4(CT3)
  [in14] -> M160/5(F3)
  [in15] -> M160/6(E3)
  [in17] -> M160/7(T3)
  [in18] -> M160/8(EB3)
  M160/1(LL2) -> Eval159/1(In2)
  M160/2(LL3) -> Eval159/2(In3)
  Eval159/1(Out1) -> To Workspace159/1
  [in7] -> M161/1(CT2)
  [in11] -> M161/2(T2)
  [in12] -> M161/3(EB2)
  [in13] -> M161/4(CT3)
  [in14] -> M161/5(F3)
  [in15] -> M161/6(E3)
  [in17] -> M161/7(T3)
  [in18] -> M161/8(EB3)
  M161/1(LL2) -> Eval160/1(In2)
  M161/2(LL3) -> Eval160/2(In3)
  Eval160/1(Out1) -> To Workspace160/1
  [in7] -> M162/1(CT2)
  [in11] -> M162/2(T2)
  [in12] -> M162/3(EB2)
  [in13] -> M162/4(CT3)
  [in14] -> M162/5(F3)
  [in15] -> M162/6(E3)
  [in17] -> M162/7(T3)
  [in18] -> M162/8(EB3)
  M162/1(LL2) -> Eval161/1(In2)
  M162/2(LL3) -> Eval161/2(In3)
  Eval161/1(Out1) -> To Workspace161/1
  [in7] -> M163/1(CT2)
  [in11] -> M163/2(T2)
  [in12] -> M163/3(EB2)
  [in13] -> M163/4(CT3)
  [in14] -> M163/5(F3)
  [in15] -> M163/6(E3)
  [in17] -> M163/7(T3)
  [in18] -> M163/8(EB3)
  M163/1(LL2) -> Eval162/1(In2)
  M163/2(LL3) -> Eval162/2(In3)
  Eval162/1(Out1) -> To Workspace162/1
  [in7] -> M164/1(CT2)
  [in11] -> M164/2(T2)
  [in12] -> M164/3(EB2)
  [in13] -> M164/4(CT3)
  [in14] -> M164/5(F3)
  [in15] -> M164/6(E3)
  [in17] -> M164/7(T3)
  [in18] -> M164/8(EB3)
  M164/1(LL2) -> Eval163/1(In2)
  M164/2(LL3) -> Eval163/2(In3)
  Eval163/1(Out1) -> To Workspace163/1
  [in7] -> M165/1(CT2)
  [in11] -> M165/2(T2)
  [in12] -> M165/3(EB2)
  [in13] -> M165/4(CT3)
  [in14] -> M165/5(F3)
  [in15] -> M165/6(E3)
  [in17] -> M165/7(T3)
  [in18] -> M165/8(EB3)
  M165/1(LL2) -> Eval164/1(In2)
  M165/2(LL3) -> Eval164/2(In3)
  Eval164/1(Out1) -> To Workspace164/1
  [in7] -> M200/1(CT2)
  [in11] -> M200/2(T2)
  [in12] -> M200/3(EB2)
  [in13] -> M200/4(CT3)
  [in14] -> M200/5(F3)
  [in15] -> M200/6(E3)
  [in17] -> M200/7(T3)
  [in18] -> M200/8(EB3)
  M200/1(LL2) -> Eval199/1(In2)
  M200/2(LL3) -> Eval199/2(In3)
  Eval199/1(Out1) -> To Workspace199/1
  [in7] -> M201/1(CT2)
  [in11] -> M201/2(T2)
  [in12] -> M201/3(EB2)
  [in13] -> M201/4(CT3)
  [in14] -> M201/5(F3)
  [in15] -> M201/6(E3)
  [in17] -> M201/7(T3)
  [in18] -> M201/8(EB3)
  M201/1(LL2) -> Eval200/1(In2)
  M201/2(LL3) -> Eval200/2(In3)
  Eval200/1(Out1) -> To Workspace200/1
  [in7] -> M202/1(CT2)
  [in11] -> M202/2(T2)
  [in12] -> M202/3(EB2)
  [in13] -> M202/4(CT3)
  [in14] -> M202/5(F3)
  [in15] -> M202/6(E3)
  [in17] -> M202/7(T3)
  [in18] -> M202/8(EB3)
  M202/1(LL2) -> Eval201/1(In2)
  M202/2(LL3) -> Eval201/2(In3)
  Eval201/1(Out1) -> To Workspace201/1
  [in7] -> M203/1(CT2)
  [in11] -> M203/2(T2)
  [in12] -> M203/3(EB2)
  [in13] -> M203/4(CT3)
  [in14] -> M203/5(F3)
  [in15] -> M203/6(E3)
  [in17] -> M203/7(T3)
  [in18] -> M203/8(EB3)
  M203/1(LL2) -> Eval202/1(In2)
  M203/2(LL3) -> Eval202/2(In3)
  Eval202/1(Out1) -> To Workspace202/1
  [in7] -> M204/1(CT2)
  [in11] -> M204/2(T2)
  [in12] -> M204/3(EB2)
  [in13] -> M204/4(CT3)
  [in14] -> M204/5(F3)
  [in15] -> M204/6(E3)
  [in17] -> M204/7(T3)
  [in18] -> M204/8(EB3)
  M204/1(LL2) -> Eval203/1(In2)
  M204/2(LL3) -> Eval203/2(In3)
  Eval203/1(Out1) -> To Workspace203/1
  [in7] -> M205/1(CT2)
  [in11] -> M205/2(T2)
  [in12] -> M205/3(EB2)
  [in13] -> M205/4(CT3)
  [in14] -> M205/5(F3)
  [in15] -> M205/6(E3)
  [in17] -> M205/7(T3)
  [in18] -> M205/8(EB3)
  M205/1(LL2) -> Eval204/1(In2)
  M205/2(LL3) -> Eval204/2(In3)
  Eval204/1(Out1) -> To Workspace204/1
  [in7] -> M206/1(CT2)
  [in11] -> M206/2(T2)
  [in12] -> M206/3(EB2)
  [in13] -> M206/4(CT3)
  [in14] -> M206/5(F3)
  [in15] -> M206/6(E3)
  [in17] -> M206/7(T3)
  [in18] -> M206/8(EB3)
  M206/1(LL2) -> Eval205/1(In2)
  M206/2(LL3) -> Eval205/2(In3)
  Eval205/1(Out1) -> To Workspace205/1
  [in7] -> M207/1(CT2)
  [in11] -> M207/2(T2)
  [in12] -> M207/3(EB2)
  [in13] -> M207/4(CT3)
  [in14] -> M207/5(F3)
  [in15] -> M207/6(E3)
  [in17] -> M207/7(T3)
  [in18] -> M207/8(EB3)
  M207/1(LL2) -> Eval206/1(In2)
  M207/2(LL3) -> Eval206/2(In3)
  Eval206/1(Out1) -> To Workspace206/1
  [in7] -> M208/1(CT2)
  [in11] -> M208/2(T2)
  [in12] -> M208/3(EB2)
  [in13] -> M208/4(CT3)
  [in14] -> M208/5(F3)
  [in15] -> M208/6(E3)
  [in17] -> M208/7(T3)
  [in18] -> M208/8(EB3)
  M208/1(LL2) -> Eval207/1(In2)
  M208/2(LL3) -> Eval207/2(In3)
  Eval207/1(Out1) -> To Workspace207/1
  [in7] -> M209/1(CT2)
  [in11] -> M209/2(T2)
  [in12] -> M209/3(EB2)
  [in13] -> M209/4(CT3)
  [in14] -> M209/5(F3)
  [in15] -> M209/6(E3)
  [in17] -> M209/7(T3)
  [in18] -> M209/8(EB3)
  M209/1(LL2) -> Eval208/1(In2)
  M209/2(LL3) -> Eval208/2(In3)
  Eval208/1(Out1) -> To Workspace208/1
  [in7] -> M222/1(CT2)
  [in11] -> M222/2(T2)
  [in12] -> M222/3(EB2)
  [in13] -> M222/4(CT3)
  [in14] -> M222/5(F3)
  [in15] -> M222/6(E3)
  [in17] -> M222/7(T3)
  [in18] -> M222/8(EB3)
  M222/1(LL2) -> Eval221/1(In2)
  M222/2(LL3) -> Eval221/2(In3)
  Eval221/1(Out1) -> To Workspace221/1
  [in7] -> M223/1(CT2)
  [in11] -> M223/2(T2)
  [in12] -> M223/3(EB2)
  [in13] -> M223/4(CT3)
  [in14] -> M223/5(F3)
  [in15] -> M223/6(E3)
  [in17] -> M223/7(T3)
  [in18] -> M223/8(EB3)
  M223/1(LL2) -> Eval222/1(In2)
  M223/2(LL3) -> Eval222/2(In3)
  Eval222/1(Out1) -> To Workspace222/1
  [in7] -> M224/1(CT2)
  [in11] -> M224/2(T2)
  [in12] -> M224/3(EB2)
  [in13] -> M224/4(CT3)
  [in14] -> M224/5(F3)
  [in15] -> M224/6(E3)
  [in17] -> M224/7(T3)
  [in18] -> M224/8(EB3)
  M224/1(LL2) -> Eval223/1(In2)
  M224/2(LL3) -> Eval223/2(In3)
  Eval223/1(Out1) -> To Workspace223/1
  [in7] -> M225/1(CT2)
  [in11] -> M225/2(T2)
  [in12] -> M225/3(EB2)
  [in13] -> M225/4(CT3)
  [in14] -> M225/5(F3)
  [in15] -> M225/6(E3)
  [in17] -> M225/7(T3)
  [in18] -> M225/8(EB3)
  M225/1(LL2) -> Eval224/1(In2)
  M225/2(LL3) -> Eval224/2(In3)
  Eval224/1(Out1) -> To Workspace224/1
  [in7] -> M226/1(CT2)
  [in11] -> M226/2(T2)
  [in12] -> M226/3(EB2)
  [in13] -> M226/4(CT3)
  [in14] -> M226/5(F3)
  [in15] -> M226/6(E3)
  [in17] -> M226/7(T3)
  [in18] -> M226/8(EB3)
  M226/1(LL2) -> Eval225/1(In2)
  M226/2(LL3) -> Eval225/2(In3)
  Eval225/1(Out1) -> To Workspace225/1
  [in7] -> M227/1(CT2)
  [in11] -> M227/2(T2)
  [in12] -> M227/3(EB2)
  [in13] -> M227/4(CT3)
  [in14] -> M227/5(F3)
  [in15] -> M227/6(E3)
  [in17] -> M227/7(T3)
  [in18] -> M227/8(EB3)
  M227/1(LL2) -> Eval226/1(In2)
  M227/2(LL3) -> Eval226/2(In3)
  Eval226/1(Out1) -> To Workspace226/1
  [in7] -> M228/1(CT2)
  [in11] -> M228/2(T2)
  [in12] -> M228/3(EB2)
  [in13] -> M228/4(CT3)
  [in14] -> M228/5(F3)
  [in15] -> M228/6(E3)
  [in17] -> M228/7(T3)
  [in18] -> M228/8(EB3)
  M228/1(LL2) -> Eval227/1(In2)
  M228/2(LL3) -> Eval227/2(In3)
  Eval227/1(Out1) -> To Workspace227/1
  [in7] -> M229/1(CT2)
  [in11] -> M229/2(T2)
  [in12] -> M229/3(EB2)
  [in13] -> M229/4(CT3)
  [in14] -> M229/5(F3)
  [in15] -> M229/6(E3)
  [in17] -> M229/7(T3)
  [in18] -> M229/8(EB3)
  M229/1(LL2) -> Eval228/1(In2)
  M229/2(LL3) -> Eval228/2(In3)
  Eval228/1(Out1) -> To Workspace228/1
  [in7] -> M230/1(CT2)
  [in11] -> M230/2(T2)
  [in12] -> M230/3(EB2)
  [in13] -> M230/4(CT3)
  [in14] -> M230/5(F3)
  [in15] -> M230/6(E3)
  [in17] -> M230/7(T3)
  [in18] -> M230/8(EB3)
  M230/1(LL2) -> Eval229/1(In2)
  M230/2(LL3) -> Eval229/2(In3)
  Eval229/1(Out1) -> To Workspace229/1
  [in7] -> M231/1(CT2)
  [in11] -> M231/2(T2)
  [in12] -> M231/3(EB2)
  [in13] -> M231/4(CT3)
  [in14] -> M231/5(F3)
  [in15] -> M231/6(E3)
  [in17] -> M231/7(T3)
  [in18] -> M231/8(EB3)
  M231/1(LL2) -> Eval230/1(In2)
  M231/2(LL3) -> Eval230/2(In3)
  Eval230/1(Out1) -> To Workspace230/1
  [in7] -> M232/1(CT2)
  [in11] -> M232/2(T2)
  [in12] -> M232/3(EB2)
  [in13] -> M232/4(CT3)
  [in14] -> M232/5(F3)
  [in15] -> M232/6(E3)
  [in17] -> M232/7(T3)
  [in18] -> M232/8(EB3)
  M232/1(LL2) -> Eval231/1(In2)
  M232/2(LL3) -> Eval231/2(In3)
  Eval231/1(Out1) -> To Workspace231/1
  [in7] -> M233/1(CT2)
  [in11] -> M233/2(T2)
  [in12] -> M233/3(EB2)
  [in13] -> M233/4(CT3)
  [in14] -> M233/5(F3)
  [in15] -> M233/6(E3)
  [in17] -> M233/7(T3)
  [in18] -> M233/8(EB3)
  M233/1(LL2) -> Eval232/1(In2)
  M233/2(LL3) -> Eval232/2(In3)
  Eval232/1(Out1) -> To Workspace232/1
  [in7] -> M234/1(CT2)
  [in11] -> M234/2(T2)
  [in12] -> M234/3(EB2)
  [in13] -> M234/4(CT3)
  [in14] -> M234/5(F3)
  [in15] -> M234/6(E3)
  [in17] -> M234/7(T3)
  [in18] -> M234/8(EB3)
  M234/1(LL2) -> Eval233/1(In2)
  M234/2(LL3) -> Eval233/2(In3)
  Eval233/1(Out1) -> To Workspace233/1
  [in7] -> M235/1(CT2)
  [in11] -> M235/2(T2)
  [in12] -> M235/3(EB2)
  [in13] -> M235/4(CT3)
  [in14] -> M235/5(F3)
  [in15] -> M235/6(E3)
  [in17] -> M235/7(T3)
  [in18] -> M235/8(EB3)
  M235/1(LL2) -> Eval234/1(In2)
  M235/2(LL3) -> Eval234/2(In3)
  Eval234/1(Out1) -> To Workspace234/1
  [in7] -> M236/1(CT2)
  [in11] -> M236/2(T2)
  [in12] -> M236/3(EB2)
  [in13] -> M236/4(CT3)
  [in14] -> M236/5(F3)
  [in15] -> M236/6(E3)
  [in17] -> M236/7(T3)
  [in18] -> M236/8(EB3)
  M236/1(LL2) -> Eval235/1(In2)
  M236/2(LL3) -> Eval235/2(In3)
  Eval235/1(Out1) -> To Workspace235/1
  [in7] -> M237/1(CT2)
  [in11] -> M237/2(T2)
  [in12] -> M237/3(EB2)
  [in13] -> M237/4(CT3)
  [in14] -> M237/5(F3)
  [in15] -> M237/6(E3)
  [in17] -> M237/7(T3)
  [in18] -> M237/8(EB3)
  M237/1(LL2) -> Eval236/1(In2)
  M237/2(LL3) -> Eval236/2(In3)
  Eval236/1(Out1) -> To Workspace236/1
  [in7] -> M238/1(CT2)
  [in11] -> M238/2(T2)
  [in12] -> M238/3(EB2)
  [in13] -> M238/4(CT3)
  [in14] -> M238/5(F3)
  [in15] -> M238/6(E3)
  [in17] -> M238/7(T3)
  [in18] -> M238/8(EB3)
  M238/1(LL2) -> Eval237/1(In2)
  M238/2(LL3) -> Eval237/2(In3)
  Eval237/1(Out1) -> To Workspace237/1
  [in7] -> M239/1(CT2)
  [in11] -> M239/2(T2)
  [in12] -> M239/3(EB2)
  [in13] -> M239/4(CT3)
  [in14] -> M239/5(F3)
  [in15] -> M239/6(E3)
  [in17] -> M239/7(T3)
  [in18] -> M239/8(EB3)
  M239/1(LL2) -> Eval238/1(In2)
  M239/2(LL3) -> Eval238/2(In3)
  Eval238/1(Out1) -> To Workspace238/1
  [in7] -> M240/1(CT2)
  [in11] -> M240/2(T2)
  [in12] -> M240/3(EB2)
  [in13] -> M240/4(CT3)
  [in14] -> M240/5(F3)
  [in15] -> M240/6(E3)
  [in17] -> M240/7(T3)
  [in18] -> M240/8(EB3)
  M240/1(LL2) -> Eval239/1(In2)
  M240/2(LL3) -> Eval239/2(In3)
  Eval239/1(Out1) -> To Workspace239/1
  [in7] -> M241/1(CT2)
  [in11] -> M241/2(T2)
  [in12] -> M241/3(EB2)
  [in13] -> M241/4(CT3)
  [in14] -> M241/5(F3)
  [in15] -> M241/6(E3)
  [in17] -> M241/7(T3)
  [in18] -> M241/8(EB3)
  M241/1(LL2) -> Eval240/1(In2)
  M241/2(LL3) -> Eval240/2(In3)
  Eval240/1(Out1) -> To Workspace240/1
  [in7] -> M242/1(CT2)
  [in11] -> M242/2(T2)
  [in12] -> M242/3(EB2)
  [in13] -> M242/4(CT3)
  [in14] -> M242/5(F3)
  [in15] -> M242/6(E3)
  [in17] -> M242/7(T3)
  [in18] -> M242/8(EB3)
  M242/1(LL2) -> Eval241/1(In2)
  M242/2(LL3) -> Eval241/2(In3)
  Eval241/1(Out1) -> To Workspace241/1
  [in7] -> M243/1(CT2)
  [in11] -> M243/2(T2)
  [in12] -> M243/3(EB2)
  [in13] -> M243/4(CT3)
  [in14] -> M243/5(F3)
  [in15] -> M243/6(E3)
  [in17] -> M243/7(T3)
  [in18] -> M243/8(EB3)
  M243/1(LL2) -> Eval242/1(In2)
  M243/2(LL3) -> Eval242/2(In3)
  Eval242/1(Out1) -> To Workspace242/1
  [in7] -> M244/1(CT2)
  [in11] -> M244/2(T2)
  [in12] -> M244/3(EB2)
  [in13] -> M244/4(CT3)
  [in14] -> M244/5(F3)
  [in15] -> M244/6(E3)
  [in17] -> M244/7(T3)
  [in18] -> M244/8(EB3)
  M244/1(LL2) -> Eval243/1(In2)
  M244/2(LL3) -> Eval243/2(In3)
  Eval243/1(Out1) -> To Workspace243/1
  [in7] -> M245/1(CT2)
  [in11] -> M245/2(T2)
  [in12] -> M245/3(EB2)
  [in13] -> M245/4(CT3)
  [in14] -> M245/5(F3)
  [in15] -> M245/6(E3)
  [in17] -> M245/7(T3)
  [in18] -> M245/8(EB3)
  M245/1(LL2) -> Eval244/1(In2)
  M245/2(LL3) -> Eval244/2(In3)
  Eval244/1(Out1) -> To Workspace244/1
  [in7] -> M246/1(CT2)
  [in11] -> M246/2(T2)
  [in12] -> M246/3(EB2)
  [in13] -> M246/4(CT3)
  [in14] -> M246/5(F3)
  [in15] -> M246/6(E3)
  [in17] -> M246/7(T3)
  [in18] -> M246/8(EB3)
  M246/1(LL2) -> Eval245/1(In2)
  M246/2(LL3) -> Eval245/2(In3)
  Eval245/1(Out1) -> To Workspace245/1
  Inputs/1(CT2) -> dtc_CT2/1
  dtc_CT2/1 -> CPSUT/1(CT2), [in7]
  Inputs/2(T2) -> dtc_T2/1
  dtc_T2/1 -> CPSUT/2(T2), [in11]
  Inputs/3(EB2) -> dtc_EB2/1
  dtc_EB2/1 -> CPSUT/3(EB2), [in12]
  Inputs/4(CT3) -> dtc_CT3/1
  dtc_CT3/1 -> CPSUT/4(CT3), [in13]
  Inputs/5(F3) -> dtc_F3/1
  dtc_F3/1 -> CPSUT/5(F3), [in14]
  Inputs/6(E3) -> dtc_E3/1
  dtc_E3/1 -> CPSUT/6(E3), [in15]
  Inputs/7(T3) -> dtc_T3/1
  dtc_T3/1 -> CPSUT/7(T3), [in17]
  Inputs/8(EB3) -> dtc_EB3/1
  dtc_EB3/1 -> CPSUT/8(EB3), [in18]

== system c00016M_harness/CPSUT ==
  note: VALUES
      | ---------------------------------
      | ControlType = 1 | 2 | 3
      | FillTank = 0 | 1
      | EmptyTank = 0 | 1
      | ManualReference between 0 and 1
      | Tempreature between 0 and 100
      | EmergencyButton = 0 | 1
      | LiquidLevel between 0 and 1 (hmax)
  note: Inputs For Tank2
  note: NAMES
      | --------------------------------------------
      | CT1 = ControlType Tank 1
      | F1 = Fill Tank 1
      | E1 = Empty Tank 1
      | MR1 = Manual Reference Tank1
      | T1 = Temperature Tank 1
      | EB1 = Emergency Button Tank 1
      | LL1 = Liquid Level 1
  note: Inputs For Tank3
  note: Inputs For Tank1
  CT2 : Inport
  T2 : Inport  Port=2
  EB2 : Inport  Port=3
  CT3 : Inport  Port=4
  F3 : Inport  Port=5
  E3 : Inport  Port=6
  T3 : Inport  Port=7
  EB3 : Inport  Port=8
  Tank2 : Subsystem
  Tank3 : Subsystem
  LL2 : Outport
  LL3 : Outport  Port=2
  wires:
  Tank2/1(LL2) -> LL2/1, Tank3/6(LL2)
  Tank3/1(LL3) -> LL3/1, Tank2/4(LL3)
  EB2/1 -> Tank2/3(EB2)
  CT2/1 -> Tank2/1(CT2)
  E3/1 -> Tank3/3(E3)
  T2/1 -> Tank2/2(T2)
  CT3/1 -> Tank3/1(CT3)
  F3/1 -> Tank3/2(F3)
  EB3/1 -> Tank3/5(EB3)
  T3/1 -> Tank3/4(T3)

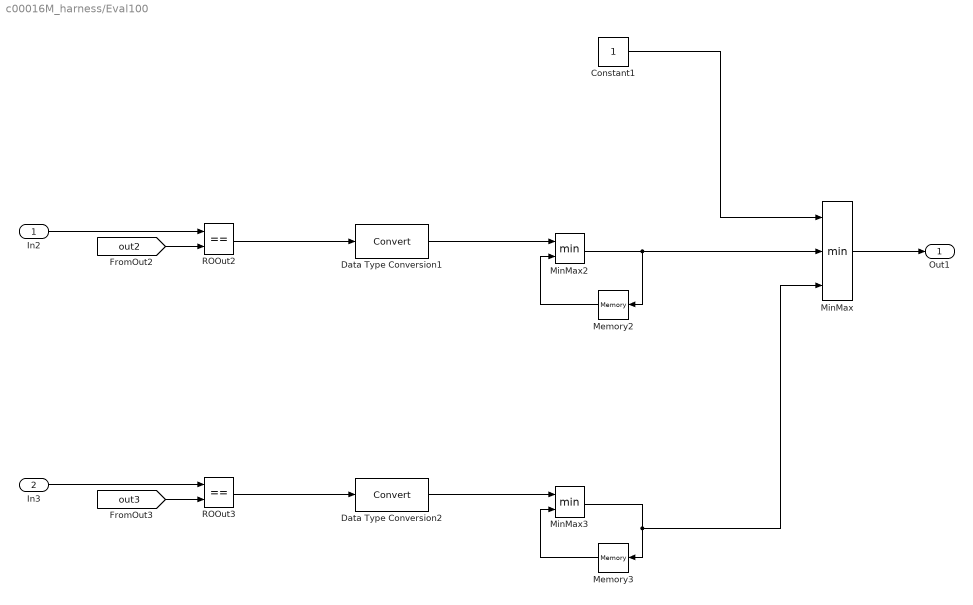
== system c00016M_harness/Eval100 ==
  In2 : Inport
  In3 : Inport  Port=2
  Constant1 : Constant
  Data Type Conversion1 : DataTypeConversion
  Data Type Conversion2 : DataTypeConversion
  Memory2 : Memory  InitialCondition=1
  Memory3 : Memory  InitialCondition=1
  MinMax : MinMax  Inputs=3
  MinMax2 : MinMax  Inputs=2
  MinMax3 : MinMax  Inputs=2
  ROOut2 : RelationalOperator  Operator===  OutDataTypeStr=boolean  RndMeth=Simplest
  ROOut3 : RelationalOperator  Operator===  OutDataTypeStr=boolean  RndMeth=Simplest
  Out1 : Outport
  wires:
  Data Type Conversion2/1 -> MinMax3/1
  Data Type Conversion1/1 -> MinMax2/1
  MinMax2/1 -> MinMax/2, Memory2/1
  Memory2/1 -> MinMax2/2
  Memory3/1 -> MinMax3/2
  ROOut2/1 -> Data Type Conversion1/1
  ROOut3/1 -> Data Type Conversion2/1
  MinMax3/1 -> Memory3/1, MinMax/3
  [out2] -> ROOut2/2
  In2/1 -> ROOut2/1
  In3/1 -> ROOut3/1
  [out3] -> ROOut3/2
  MinMax/1 -> Out1/1
  Constant1/1 -> MinMax/1

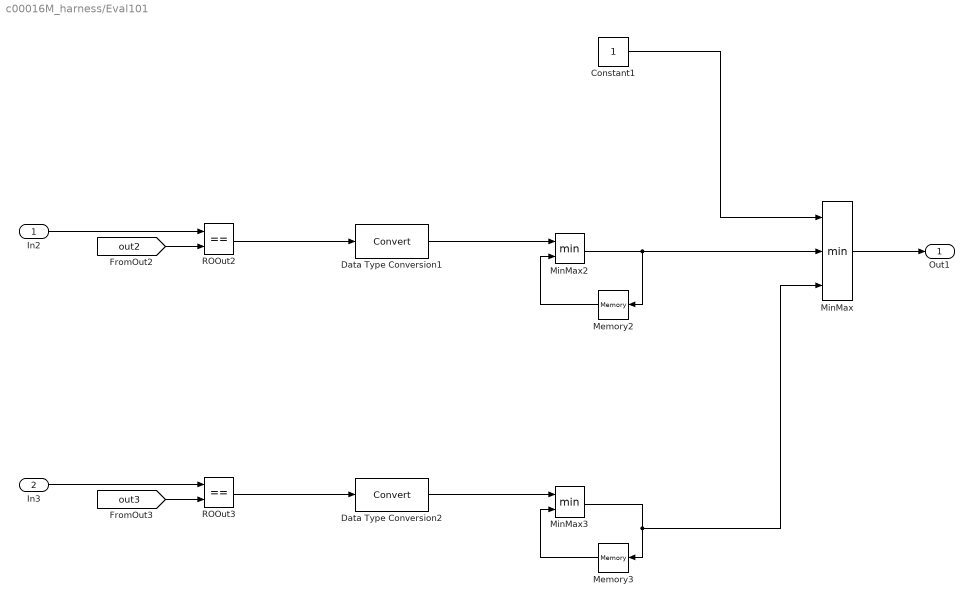
== system c00016M_harness/Eval101 ==
  In2 : Inport
  In3 : Inport  Port=2
  Constant1 : Constant
  Data Type Conversion1 : DataTypeConversion
  Data Type Conversion2 : DataTypeConversion
  Memory2 : Memory  InitialCondition=1
  Memory3 : Memory  InitialCondition=1
  MinMax : MinMax  Inputs=3
  MinMax2 : MinMax  Inputs=2
  MinMax3 : MinMax  Inputs=2
  ROOut2 : RelationalOperator  Operator===  OutDataTypeStr=boolean  RndMeth=Simplest
  ROOut3 : RelationalOperator  Operator===  OutDataTypeStr=boolean  RndMeth=Simplest
  Out1 : Outport
  wires:
  Data Type Conversion2/1 -> MinMax3/1
  Data Type Conversion1/1 -> MinMax2/1
  MinMax2/1 -> MinMax/2, Memory2/1
  Memory2/1 -> MinMax2/2
  Memory3/1 -> MinMax3/2
  ROOut2/1 -> Data Type Conversion1/1
  ROOut3/1 -> Data Type Conversion2/1
  MinMax3/1 -> Memory3/1, MinMax/3
  [out2] -> ROOut2/2
  In2/1 -> ROOut2/1
  In3/1 -> ROOut3/1
  [out3] -> ROOut3/2
  MinMax/1 -> Out1/1
  Constant1/1 -> MinMax/1

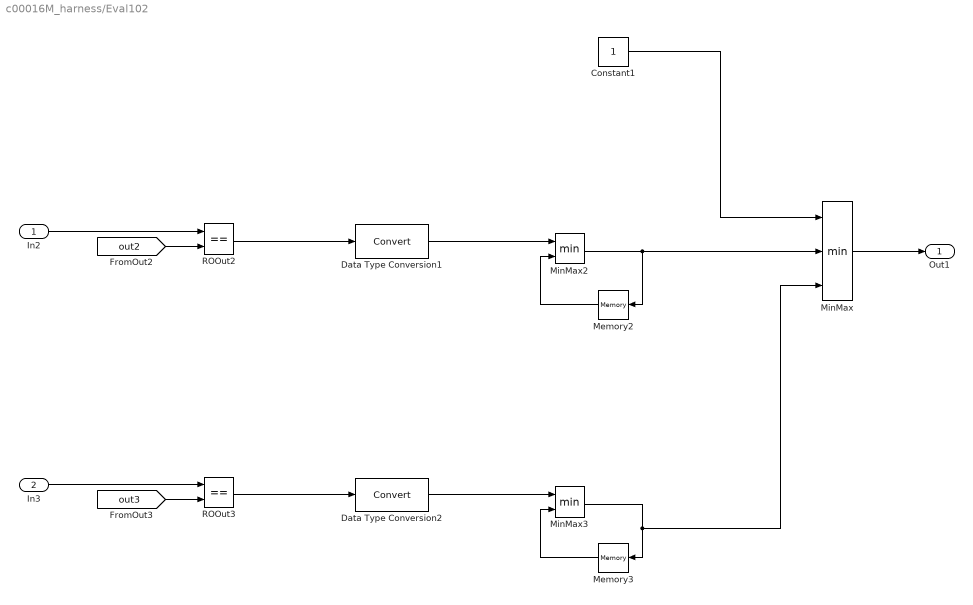
== system c00016M_harness/Eval102 ==
  In2 : Inport
  In3 : Inport  Port=2
  Constant1 : Constant
  Data Type Conversion1 : DataTypeConversion
  Data Type Conversion2 : DataTypeConversion
  Memory2 : Memory  InitialCondition=1
  Memory3 : Memory  InitialCondition=1
  MinMax : MinMax  Inputs=3
  MinMax2 : MinMax  Inputs=2
  MinMax3 : MinMax  Inputs=2
  ROOut2 : RelationalOperator  Operator===  OutDataTypeStr=boolean  RndMeth=Simplest
  ROOut3 : RelationalOperator  Operator===  OutDataTypeStr=boolean  RndMeth=Simplest
  Out1 : Outport
  wires:
  Data Type Conversion2/1 -> MinMax3/1
  Data Type Conversion1/1 -> MinMax2/1
  MinMax2/1 -> MinMax/2, Memory2/1
  Memory2/1 -> MinMax2/2
  Memory3/1 -> MinMax3/2
  ROOut2/1 -> Data Type Conversion1/1
  ROOut3/1 -> Data Type Conversion2/1
  MinMax3/1 -> Memory3/1, MinMax/3
  [out2] -> ROOut2/2
  In2/1 -> ROOut2/1
  In3/1 -> ROOut3/1
  [out3] -> ROOut3/2
  MinMax/1 -> Out1/1
  Constant1/1 -> MinMax/1

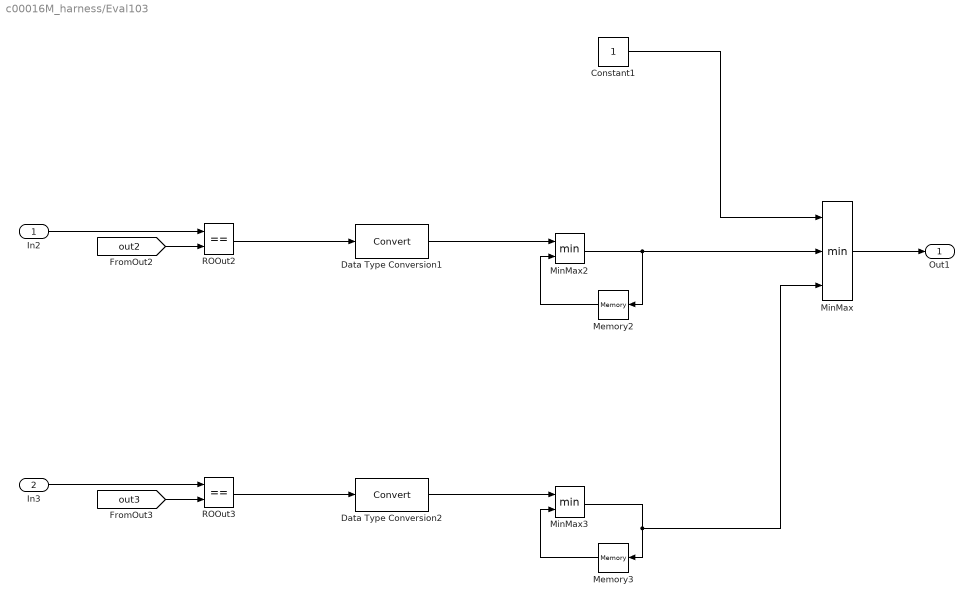
== system c00016M_harness/Eval103 ==
  In2 : Inport
  In3 : Inport  Port=2
  Constant1 : Constant
  Data Type Conversion1 : DataTypeConversion
  Data Type Conversion2 : DataTypeConversion
  Memory2 : Memory  InitialCondition=1
  Memory3 : Memory  InitialCondition=1
  MinMax : MinMax  Inputs=3
  MinMax2 : MinMax  Inputs=2
  MinMax3 : MinMax  Inputs=2
  ROOut2 : RelationalOperator  Operator===  OutDataTypeStr=boolean  RndMeth=Simplest
  ROOut3 : RelationalOperator  Operator===  OutDataTypeStr=boolean  RndMeth=Simplest
  Out1 : Outport
  wires:
  Data Type Conversion2/1 -> MinMax3/1
  Data Type Conversion1/1 -> MinMax2/1
  MinMax2/1 -> MinMax/2, Memory2/1
  Memory2/1 -> MinMax2/2
  Memory3/1 -> MinMax3/2
  ROOut2/1 -> Data Type Conversion1/1
  ROOut3/1 -> Data Type Conversion2/1
  MinMax3/1 -> Memory3/1, MinMax/3
  [out2] -> ROOut2/2
  In2/1 -> ROOut2/1
  In3/1 -> ROOut3/1
  [out3] -> ROOut3/2
  MinMax/1 -> Out1/1
  Constant1/1 -> MinMax/1

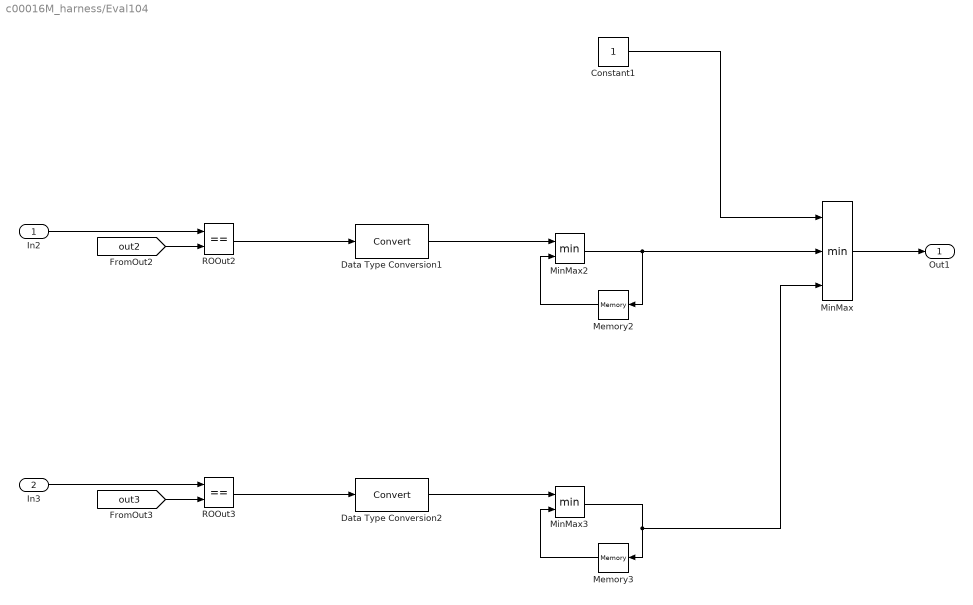
== system c00016M_harness/Eval104 ==
  In2 : Inport
  In3 : Inport  Port=2
  Constant1 : Constant
  Data Type Conversion1 : DataTypeConversion
  Data Type Conversion2 : DataTypeConversion
  Memory2 : Memory  InitialCondition=1
  Memory3 : Memory  InitialCondition=1
  MinMax : MinMax  Inputs=3
  MinMax2 : MinMax  Inputs=2
  MinMax3 : MinMax  Inputs=2
  ROOut2 : RelationalOperator  Operator===  OutDataTypeStr=boolean  RndMeth=Simplest
  ROOut3 : RelationalOperator  Operator===  OutDataTypeStr=boolean  RndMeth=Simplest
  Out1 : Outport
  wires:
  Data Type Conversion2/1 -> MinMax3/1
  Data Type Conversion1/1 -> MinMax2/1
  MinMax2/1 -> MinMax/2, Memory2/1
  Memory2/1 -> MinMax2/2
  Memory3/1 -> MinMax3/2
  ROOut2/1 -> Data Type Conversion1/1
  ROOut3/1 -> Data Type Conversion2/1
  MinMax3/1 -> Memory3/1, MinMax/3
  [out2] -> ROOut2/2
  In2/1 -> ROOut2/1
  In3/1 -> ROOut3/1
  [out3] -> ROOut3/2
  MinMax/1 -> Out1/1
  Constant1/1 -> MinMax/1

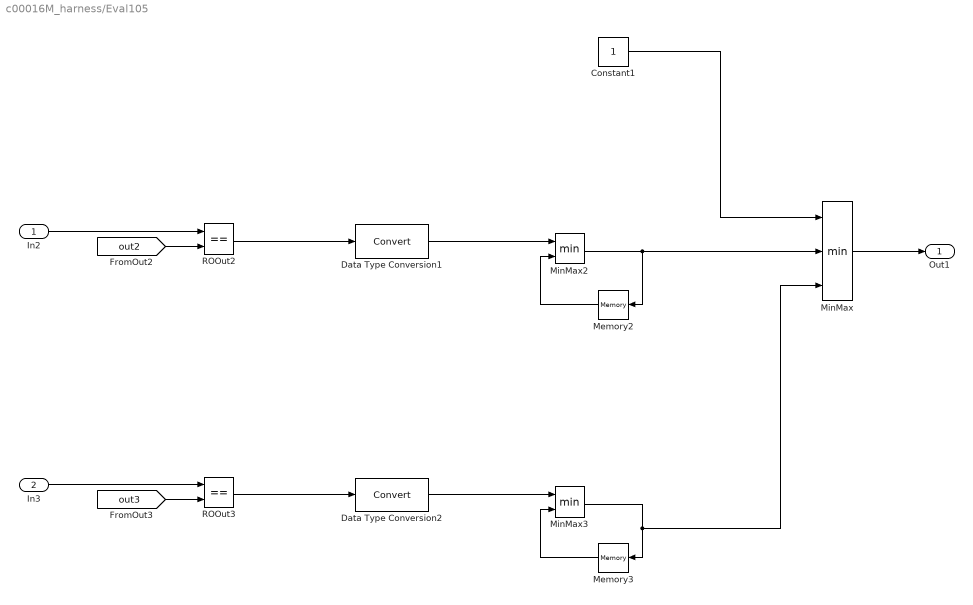
== system c00016M_harness/Eval105 ==
  In2 : Inport
  In3 : Inport  Port=2
  Constant1 : Constant
  Data Type Conversion1 : DataTypeConversion
  Data Type Conversion2 : DataTypeConversion
  Memory2 : Memory  InitialCondition=1
  Memory3 : Memory  InitialCondition=1
  MinMax : MinMax  Inputs=3
  MinMax2 : MinMax  Inputs=2
  MinMax3 : MinMax  Inputs=2
  ROOut2 : RelationalOperator  Operator===  OutDataTypeStr=boolean  RndMeth=Simplest
  ROOut3 : RelationalOperator  Operator===  OutDataTypeStr=boolean  RndMeth=Simplest
  Out1 : Outport
  wires:
  Data Type Conversion2/1 -> MinMax3/1
  Data Type Conversion1/1 -> MinMax2/1
  MinMax2/1 -> MinMax/2, Memory2/1
  Memory2/1 -> MinMax2/2
  Memory3/1 -> MinMax3/2
  ROOut2/1 -> Data Type Conversion1/1
  ROOut3/1 -> Data Type Conversion2/1
  MinMax3/1 -> Memory3/1, MinMax/3
  [out2] -> ROOut2/2
  In2/1 -> ROOut2/1
  In3/1 -> ROOut3/1
  [out3] -> ROOut3/2
  MinMax/1 -> Out1/1
  Constant1/1 -> MinMax/1

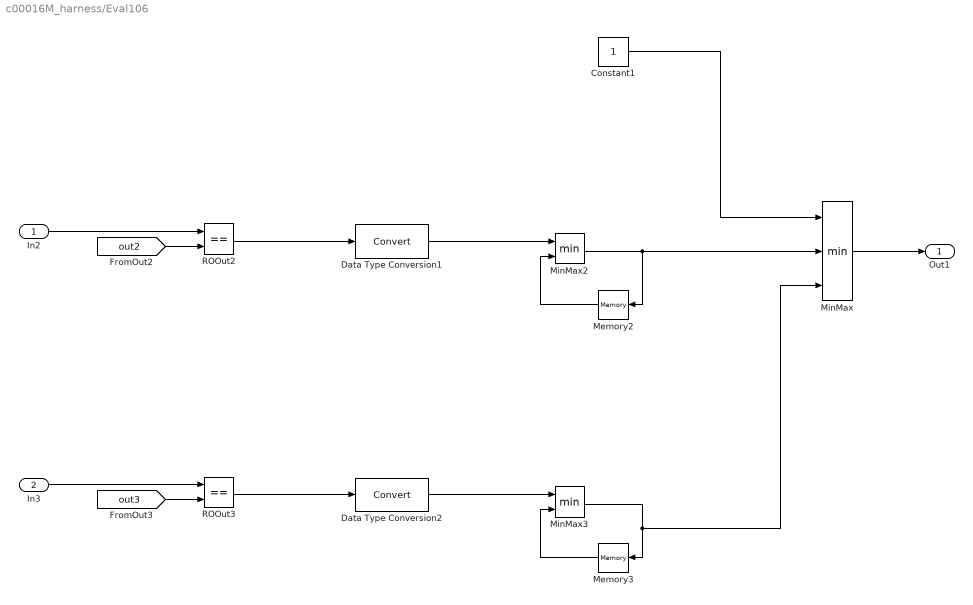
== system c00016M_harness/Eval106 ==
  In2 : Inport
  In3 : Inport  Port=2
  Constant1 : Constant
  Data Type Conversion1 : DataTypeConversion
  Data Type Conversion2 : DataTypeConversion
  Memory2 : Memory  InitialCondition=1
  Memory3 : Memory  InitialCondition=1
  MinMax : MinMax  Inputs=3
  MinMax2 : MinMax  Inputs=2
  MinMax3 : MinMax  Inputs=2
  ROOut2 : RelationalOperator  Operator===  OutDataTypeStr=boolean  RndMeth=Simplest
  ROOut3 : RelationalOperator  Operator===  OutDataTypeStr=boolean  RndMeth=Simplest
  Out1 : Outport
  wires:
  Data Type Conversion2/1 -> MinMax3/1
  Data Type Conversion1/1 -> MinMax2/1
  MinMax2/1 -> MinMax/2, Memory2/1
  Memory2/1 -> MinMax2/2
  Memory3/1 -> MinMax3/2
  ROOut2/1 -> Data Type Conversion1/1
  ROOut3/1 -> Data Type Conversion2/1
  MinMax3/1 -> Memory3/1, MinMax/3
  [out2] -> ROOut2/2
  In2/1 -> ROOut2/1
  In3/1 -> ROOut3/1
  [out3] -> ROOut3/2
  MinMax/1 -> Out1/1
  Constant1/1 -> MinMax/1
